simulink model "koyz1"  (R2021a)
settings: Solver=FixedStepDiscrete  StartTime=0.0  StopTime=512  RelTol=1e-3
libraries: dspxfrm3 x1, dspsrcs4 x1
settings Model: Creator=User1  LastModifiedBy=User1

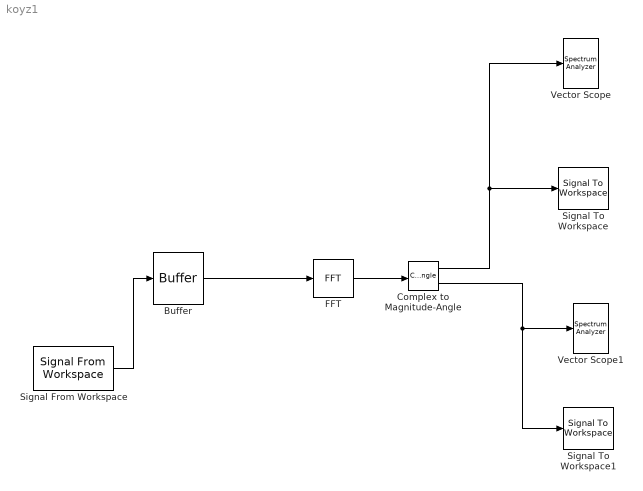
== system koyz1 ==
  Buffer : Buffer  N=512
  Complex to Magnitude-Angle : ComplexToMagnitudeAngle
  FFT : dspxfrm3/FFT  FFTImplementation=Auto  CompMethod=Table lookup  TableOpt=NEW  TableOptActive=Speed  BitRevOrder=off  Normalize=off  InheritFFTLength=on  FFTLength=64  WrapInput=on  roundingMode=Floor  overflowMode=off  firstCoeffDataTypeStr=Inherit: Same word length as input  firstCoeffLastDataTypeStr=Inherit: Same word length as input  outputMin=[]  outputMax=[]
  Signal From Workspace : dspsrcs4/Signal From Workspace  X=[5 8 6 5 0 1 9]  Ts=1  nsamps=1  OutputAfterFinalValue=Setting to zero  ignoreOrWarnInputAndFrameLengths=off  OutputFrames=on
  Signal To Workspace : SignalToWorkspace  VariableName=mag
      settings: CopyFcn=dspblkcopystw(gcbh);
  Signal To Workspace1 : SignalToWorkspace  VariableName=phase
      settings: CopyFcn=dspblkcopystw(gcbh);
  Vector Scope : SpectrumAnalyzer
  Vector Scope1 : SpectrumAnalyzer
  wires:
  Buffer/1 -> FFT/1
  Complex to Magnitude-Angle/1 -> Signal To Workspace/1, Vector Scope/1
  FFT/1 -> Complex to Magnitude-Angle/1
  Complex to Magnitude-Angle/2 -> Vector Scope1/1, Signal To Workspace1/1
  Signal From Workspace/1 -> Buffer/1
